simulink model "Comparison_to_Nest_Neuron"  (R2020b)
settings: Solver=VariableStepAuto  StartTime=0.0  StopTime=0.4  RelTol=1e-3
libraries: NeuroModelerLibrary x3
settings Model: Creator=Александра  LastModifiedBy=Александра

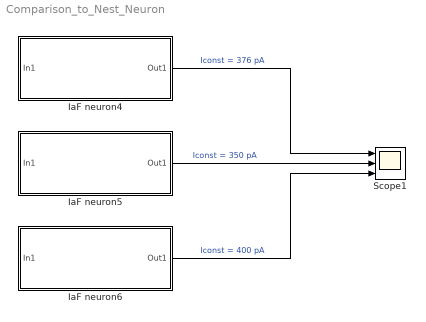
== system Comparison_to_Nest_Neuron ==
  IaF neuron4 : Subsystem  mask{tau_m=0.010, Cm=250e-12, I_const=376e-12, E_L=-0.070, V_reset=-0.070, V_th=-0.055}
      mask prompts: tau_m "Membrane time constatnt"; Cm "Membrane capacity"; I_const "Constant input current"; E_L "Resting membrane potential"; V_reset "Reset membrane potential"; V_th "Threshold potential"
  IaF neuron5 : Subsystem  mask{tau_m=0.010, Cm=250e-12, I_const=350e-12, E_L=-0.070, V_reset=-0.070, V_th=-0.055}
      mask prompts: tau_m "Membrane time constatnt"; Cm "Membrane capacity"; I_const "Constant input current"; E_L "Resting membrane potential"; V_reset "Reset membrane potential"; V_th "Threshold potential"
  IaF neuron6 : Subsystem  mask{tau_m=0.010, Cm=250e-12, I_const=400e-12, E_L=-0.070, V_reset=-0.070, V_th=-0.055}
      mask prompts: tau_m "Membrane time constatnt"; Cm "Membrane capacity"; I_const "Constant input current"; E_L "Resting membrane potential"; V_reset "Reset membrane potential"; V_th "Threshold potential"
  Scope1 : Scope  NumInputPorts=3
  wires:
  IaF neuron4/1(Out1) -> Scope1/1  "Iconst = 376 pA"
  IaF neuron5/1(Out1) -> Scope1/2  "Iconst = 350 pA"
  IaF neuron6/1(Out1) -> Scope1/3  "Iconst = 400 pA"

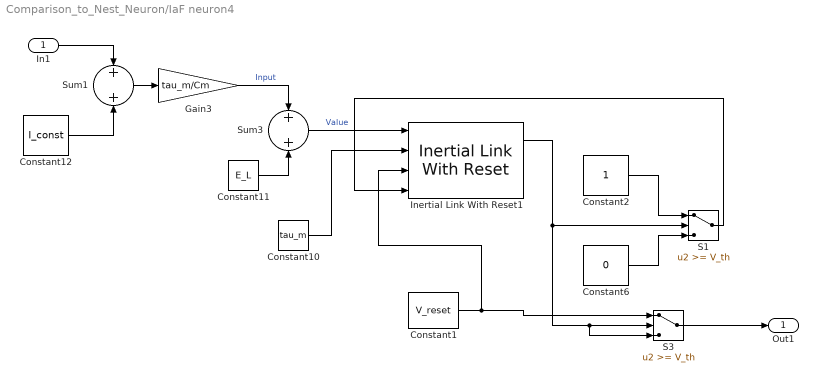
== system Comparison_to_Nest_Neuron/IaF neuron4 ==
  In1 : Inport
  Constant1 : Constant  Value=V_reset
  Constant10 : Constant  Value=tau_m
  Constant11 : Constant  Value=E_L
  Constant12 : Constant  Value=I_const
  Constant2 : Constant
  Constant6 : Constant  Value=0
  Gain3 : Gain  Gain=tau_m/Cm
  Inertial Link With Reset1 : NeuroModelerLibrary/Support/Inertial Link With Reset  SystemSampleTime=-1  VariantActivationTime=update diagram  Latency=0  AutoFrameSizeCalculation=off
  S1 : Switch  Threshold=V_th  SaturateOnIntegerOverflow=on  InputSameDT=on
  S3 : Switch  Threshold=V_th  SaturateOnIntegerOverflow=on  InputSameDT=on
  Sum1 : Sum
  Sum3 : Sum
  Out1 : Outport
  wires:
  Constant11/1 -> Sum3/2
  Constant10/1 -> Inertial Link With Reset1/2
  In1/1 -> Sum1/1
  Sum1/1 -> Gain3/1
  Constant12/1 -> Sum1/2
  Constant2/1 -> S1/1
  Constant6/1 -> S1/3
  Sum3/1 -> Inertial Link With Reset1/1  "Value"
  Inertial Link With Reset1/1 -> S1/2, S3/3, S3/2
  Constant1/1 -> Inertial Link With Reset1/3, S3/1
  S1/1 -> Inertial Link With Reset1/4
  S3/1 -> Out1/1
  Gain3/1 -> Sum3/1  "Input"

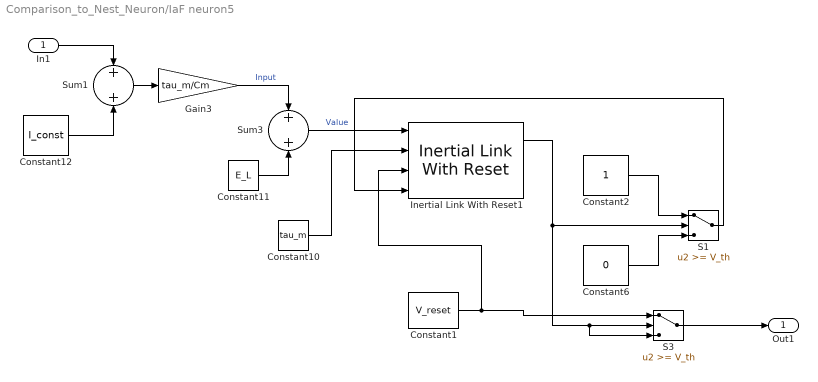
== system Comparison_to_Nest_Neuron/IaF neuron5 ==
  In1 : Inport
  Constant1 : Constant  Value=V_reset
  Constant10 : Constant  Value=tau_m
  Constant11 : Constant  Value=E_L
  Constant12 : Constant  Value=I_const
  Constant2 : Constant
  Constant6 : Constant  Value=0
  Gain3 : Gain  Gain=tau_m/Cm
  Inertial Link With Reset1 : NeuroModelerLibrary/Support/Inertial Link With Reset  SystemSampleTime=-1  VariantActivationTime=update diagram  Latency=0  AutoFrameSizeCalculation=off
  S1 : Switch  Threshold=V_th  SaturateOnIntegerOverflow=on  InputSameDT=on
  S3 : Switch  Threshold=V_th  SaturateOnIntegerOverflow=on  InputSameDT=on
  Sum1 : Sum
  Sum3 : Sum
  Out1 : Outport
  wires:
  Constant11/1 -> Sum3/2
  Constant10/1 -> Inertial Link With Reset1/2
  In1/1 -> Sum1/1
  Sum1/1 -> Gain3/1
  Constant12/1 -> Sum1/2
  Constant2/1 -> S1/1
  Constant6/1 -> S1/3
  Sum3/1 -> Inertial Link With Reset1/1  "Value"
  Inertial Link With Reset1/1 -> S1/2, S3/3, S3/2
  Constant1/1 -> Inertial Link With Reset1/3, S3/1
  S1/1 -> Inertial Link With Reset1/4
  S3/1 -> Out1/1
  Gain3/1 -> Sum3/1  "Input"

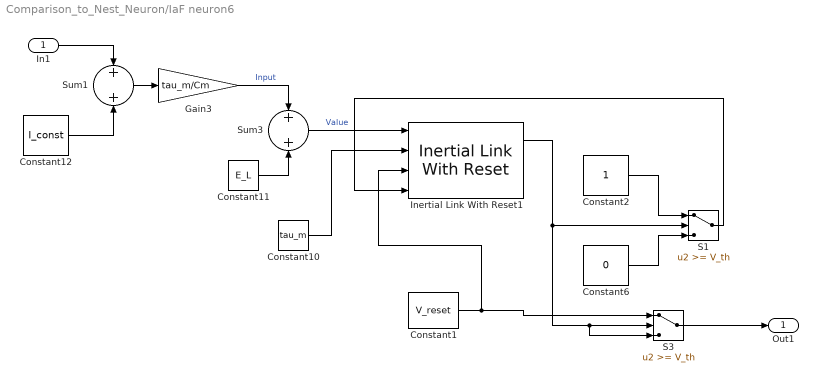
== system Comparison_to_Nest_Neuron/IaF neuron6 ==
  In1 : Inport
  Constant1 : Constant  Value=V_reset
  Constant10 : Constant  Value=tau_m
  Constant11 : Constant  Value=E_L
  Constant12 : Constant  Value=I_const
  Constant2 : Constant
  Constant6 : Constant  Value=0
  Gain3 : Gain  Gain=tau_m/Cm
  Inertial Link With Reset1 : NeuroModelerLibrary/Support/Inertial Link With Reset  SystemSampleTime=-1  VariantActivationTime=update diagram  Latency=0  AutoFrameSizeCalculation=off
  S1 : Switch  Threshold=V_th  SaturateOnIntegerOverflow=on  InputSameDT=on
  S3 : Switch  Threshold=V_th  SaturateOnIntegerOverflow=on  InputSameDT=on
  Sum1 : Sum
  Sum3 : Sum
  Out1 : Outport
  wires:
  Constant11/1 -> Sum3/2
  Constant10/1 -> Inertial Link With Reset1/2
  In1/1 -> Sum1/1
  Sum1/1 -> Gain3/1
  Constant12/1 -> Sum1/2
  Constant2/1 -> S1/1
  Constant6/1 -> S1/3
  Sum3/1 -> Inertial Link With Reset1/1  "Value"
  Inertial Link With Reset1/1 -> S1/2, S3/3, S3/2
  Constant1/1 -> Inertial Link With Reset1/3, S3/1
  S1/1 -> Inertial Link With Reset1/4
  S3/1 -> Out1/1
  Gain3/1 -> Sum3/1  "Input"
